simulink model "hyb_integral_action_model"  (Simulink 5.0)
settings: Solver=ode45  StartTime=0.0  StopTime=10.0  RelTol=1e-3
values from neighbouring files (symbols this model uses):
  HybMPC = hybcon(extended_plant,Q,N,limits,refs)    [hyb_integral_action.m]    (also in hyb_meas_dist.m)
libraries: hyblib x2
settings Model: LastModifiedBy=Alberto Bemporad  RTWOptions="-aEnforceIntegerDowncast=1 -aFoldNonRolledExpr=1 -aInlineInvariantSignals=0 -aInlineParameters=0 -aLocalBlockOutputs=1 -aRollThreshold=5 -aGenerateReport=0 -aGenCodeOnly=0 -aRTWVerbose=1 -aIncludeHyperlinkInReport=0 -aLaunchReport=0 -aForceParamTrailComments=0 -aGenerateComments=1 -aIgnoreCustomStorageClasses=1 -aIncHierarchyInIds=0 -aMaxRTWIdLen=31 -aShowEliminatedStatements=0 -aPrefixModelToSubsysFcnNames=1 -aIncDataTypeInIds=0 -aInsertBlockDesc=0 -aSimulinkBlockComments=1 -aInlinedPrmAccess=\"Literals\"  -aSuppressErrorStatus=0 -aModelReferenceCompliant=1 -aSupportNonInlinedSFcns=1 -aSupportContinuousTime=1 -aSupportComplex=1 -aSupportNonFinite=1 -aSupportAbsoluteTime=1 -aTargetPreCompLibLocation=\"\" -aTargetLibSuffix=\"\" -aTargetFcnLib=\"ansi_tfl_tmw.mat\" -aMultiInstanceERTCode=0 -aLogVarNameModifier=\"rt_\" -aIsPILTarget=0 -aCombineOutputUpdateFcns=0 -aGenerateASAP2=0 -aGenerateSampleERTMain=0 -aGenerateFullHeader=1 -aUtilityFuncGeneration=\"Auto\" -aIncludeFileDelimiter=\"Auto\" -aIncludeMdlTerminateFcn=1 -aPurelyIntegerCode=0 -aERTCustomFileBanners=0 -aRTWCAPIStates=0 -aRTWCAPIParams=0 -aRTWCAPISignals=0 -aMatFileLogging=1 -aGenFloatMathFcnCalls=\"ANSI_C\" -aExtModeMexFile=\"ext_comm\" -aExtModeTransport=0 -aExtModeStaticAllocSize=1000000 -aExtModeTesting=0 -aExtModeStaticAlloc=0 -aExtMode=0"

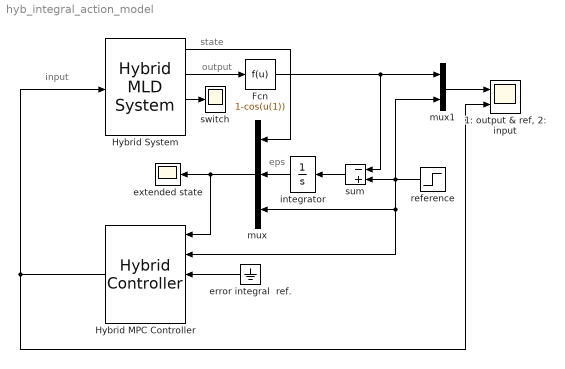
== system hyb_integral_action_model ==
  note: state
  note: output
  note: input
  note: eps
  "1: output & ref, 2: input" : Scope  NumInputPorts=2
      settings: TimeRange=10  YMin=0~0  YMax=1.5~2.5
  Fcn : Fcn  Expr=1-cos(u(1))
  Hybrid MPC Controller : hyblib/Hybrid Controller  Orientation=left  C=HybMPC  S=extended_plant
  Hybrid System : hyblib/Hybrid MLD System  S=plant  x0init=x0
  error integral  ref. : Ground  Orientation=left
  extended state : Scope
      settings: SaveName=ScopeData3
  integrator : Integrator  Orientation=left
  mux : Mux  Orientation=left  Inputs=3
  mux1 : Mux  Inputs=2
  reference : Step  Orientation=left  Time=0
  sum : Sum  Orientation=left  Inputs=-+  SaturateOnIntegerOverflow=on  InputSameDT=on
  switch : Scope
  wires:
  Hybrid MPC Controller/1 -> Hybrid System/1, "1: output & ref, 2: input"/2
  sum/1 -> integrator/1
  reference/1 -> sum/2, Hybrid MPC Controller/2, mux/3, mux1/2
  Hybrid System/2 -> Fcn/1
  mux/1 -> Hybrid MPC Controller/1, extended state/1
  Hybrid System/1 -> mux/1
  integrator/1 -> mux/2
  mux1/1 -> "1: output & ref, 2: input"/1
  Hybrid System/3 -> switch/1
  Fcn/1 -> sum/1, mux1/1
  error integral  ref./1 -> Hybrid MPC Controller/3
